simulink model "MotorModelVariable"  (R2016b)
settings: Solver=VariableStepAuto  StartTime=0.0  StopTime=10.0  RelTol=1e-3  EnableMultiTasking=on
undefined symbols (not defined in the file or in its folder): Initial, Motor, Uav
settings Model: Creator=jban039  LastModifiedBy=jban039
settings DataIOCC: LimitDataPoints=on
settings OptimizationCC: LifeSpan=inf
settings DebuggingCC: AllowSymbolicDim=off  SFUnexpectedBacktrackingDiag=warning  SFNoUnconditionalDefaultTransitionDiag=warning  SFExecutionAtInitializationDiag=none
settings ModelReferenceCC: PropagateSignalLabelsOutOfModel=off
settings GRTTargetCC: TargetLangStandard=C89/C90 (ANSI)
settings ConfigComp: CovMetricSettings=dw  CovHtmlReporting=on  CovSaveCumulativeToWorkspaceVar=on  CovSaveSingleToWorkspaceVar=on  CovExternalEMLEnable=off

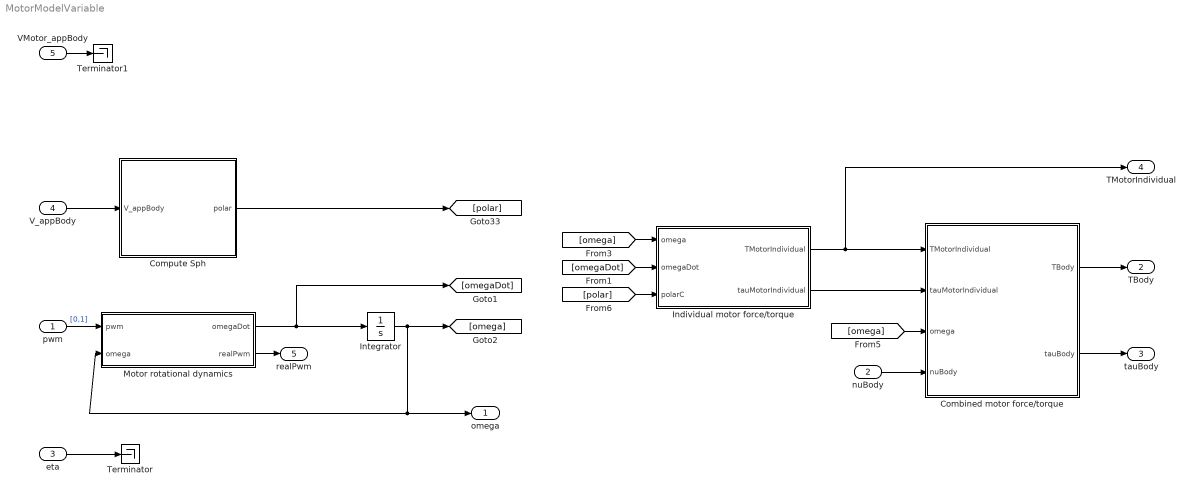
== system MotorModelVariable ==
  pwm : Inport  PortDimensions=Uav.N_ROTORS
  nuBody : Inport  Port=2  Unit=rad/s  PortDimensions=3
  eta : Inport  Port=3  Unit=rad  PortDimensions=3
  V_appBody : Inport  Port=4  Unit=m/s  PortDimensions=3
  VMotor_appBody : Inport  Port=5  Unit=m/s  PortDimensions=[3,4]
  Combined motor force/torque : MATLAB Function  TreatAsAtomicUnit=on
  Compute Sph : MATLAB Function  TreatAsAtomicUnit=on
  Individual motor force/torque : MATLAB Function  TreatAsAtomicUnit=on
  Integrator : Integrator  InitialCondition=Initial.OMEGA
  Motor rotational dynamics : MATLAB Function  TreatAsAtomicUnit=on
  Terminator : Terminator
  Terminator1 : Terminator
  omega : Outport  Unit=rad/s
  TBody : Outport  Port=2  Unit=N
  tauBody : Outport  Port=3  Unit=N*m
  TMotorIndividual : Outport  Port=4  Unit=N
  realPwm : Outport  Port=5
  wires:
  Combined motor force/torque/2(tauBody) -> tauBody/1
  Combined motor force/torque/1(TBody) -> TBody/1
  pwm/1 -> Motor rotational dynamics/1(pwm)  "[0,1]"
  eta/1 -> Terminator/1
  V_appBody/1 -> Compute Sph/1(V_appBody)
  Individual motor force/torque/2(tauMotorIndividual) -> Combined motor force/torque/2(tauMotorIndividual)
  Motor rotational dynamics/1(omegaDot) -> [omegaDot], Integrator/1
  nuBody/1 -> Combined motor force/torque/4(nuBody)
  Compute Sph/1(polar) -> [polar]
  Individual motor force/torque/1(TMotorIndividual) -> Combined motor force/torque/1(TMotorIndividual), TMotorIndividual/1
  [omegaDot] -> Individual motor force/torque/2(omegaDot)
  Integrator/1 -> [omega], Motor rotational dynamics/2(omega), omega/1
  [omega] -> Individual motor force/torque/1(omega)
  [omega] -> Combined motor force/torque/3(omega)
  [polar] -> Individual motor force/torque/3(polarC)
  Motor rotational dynamics/2(realPwm) -> realPwm/1
  VMotor_appBody/1 -> Terminator1/1

== matlab function MotorModelVariable/Compute Sph ==
  data: V_appBody input; polar output
function polar  = computeSph(V_appBody)
%#codegen

% Convert from polar to spherical coordinates

margin = 0.01;

% if ( ( V_appBody(1) < margin ) && ( V_appBody(3) < margin ) )
%     radius = sqrt( sum( V_appBody.^2 ) );
%     azimuth = 0;
%     elevation = 0;
% else
    [ azimuth, elevation, radius ] = cart2sph( V_appBody(1), V_appBody(2), V_appBody(3) );
% end



polar = [azimuth; elevation; radius];

== matlab function MotorModelVariable/Individual motor force//torque ==
  data: omega input; TMotorIndividual output size=[3 4]; omegaDot input; polarC input; Motor parameter; Uav parameter; tauMotorIndividual output size=[3 4]
function [TMotorIndividual, tauMotorIndividual] = motorIndividual( ...
    omega, omegaDot, polarC, Motor, Uav)
%#codegen

elevation = polarC(2);
windSpeed = polarC(3);

% Make assertions to avoid code generation errors
% assert(Uav.N_ROTORS < 16);
Uav.N_ROTORS = 4;

%% Thrust and differential torque

% Concatenated motor force/torque vectors in respective motor frame
% eg. TMotor = [TMotor1, TMotor2, ..., TMotorN]
% where: - N is the number of rotors
%        - TMotorx (x ∈ [1,2,...,N]) is the thrust generated by motor x in
%          its own frame of reference
% TMotorIndividual = [ zeros(2, Uav.N_ROTORS);
%                      K * (omega'.^2) ];

K1 = 6.543988868292138e-05 + ...
     1.886359198743874e-06 * sin(-elevation) + ...
    -7.693938774360465e-07 * windSpeed + ...
     2.639630950517221e-06 * sin(-elevation) * windSpeed + ...
     2.126334444415667e-08 * windSpeed^2;
K2 = -1.903771811601254e-04 + ...
      2.812570127999989e-03 * sin(-elevation) + ...
      1.418616236881443e-03 * windSpeed + ...
     -4.525882966383329e-03 * sin(-elevation) * windSpeed + ...
     -1.658875316836167e-05 * windSpeed^2;

% RECOMPUTE THRUST COEFFICIENTS AS CURRENT VALUES OUT BY FACTOR OF 4
TMotorIndividual = [ zeros(2, Uav.N_ROTORS);
                     0.25 * 0.5 * Uav.RHO_AIR * K1 * (omega'.^2) + ...
                     0.25 * 0.5 * Uav.RHO_AIR * K2 * (omega') ];
tauMotorIndividual = zeros(3, Uav.N_ROTORS);                 
for i = 1:Uav.N_ROTORS
    tauMotorIndividual(:,i) = [ zeros(2, 1);
                               -Uav.ROTOR_DIRECTION(i) .* ...
                               ( Motor.B(i) * (omega(i)'.^2) + Motor.I_R(3,3,i) * omegaDot(i)' ) ];
end

== matlab function MotorModelVariable/Motor rotational dynamics ==
  data: pwm input; omegaDot output; omega input; realPwm output
function [omegaDot, realPwm]  = motorRotDynamics( pwm, omega)
%#codegen

realPwm = (1000 * pwm + 1000);
% realPwm(2) = realPwm(2) - 200;
% realPwm(4) = realPwm(4) - 200;

% realPwm( realPwm < 1230 ) = 1230;

rotorTimeConst = 7.006512e-02;
omegaRef = zeros(4,1);
omegaRef([1 3]) = 0.87*sqrt(0.69)*(7.969173e-1 .* realPwm([1 3]) - 6.528579e2);
omegaRef([2 4]) = 0.87*sqrt(1.31)*(7.969173e-1 .* realPwm([2 4]) - 6.528579e2);
%omegaRef = 7.969173e-1 .* realPwm - 6.528579e2;

omegaDot = (omegaRef - omega) / rotorTimeConst;

== matlab function MotorModelVariable/Combined motor force//torque ==
  data: TMotorIndividual input; TBody output size=3; tauMotorIndividual input; tauBody output size=3; omega input; nuBody input; Motor parameter; Uav parameter
function [TBody, tauBody] = motorCombined( TMotorIndividual,tauMotorIndividual,  ...
    omega, nuBody, Motor, Uav)
%#codegen
assert(Uav.N_ROTORS < 16);

% Initialise matrices to store motor force/torque vectors in body frame
TBodyIndividual   = zeros(3, Uav.N_ROTORS);
tauBodyIndividual = zeros(3, Uav.N_ROTORS);

% Calculate forces and moments from each motor in the body frame
for i = 1:Uav.N_ROTORS
    l = Uav.L(i);
    beta = Uav.BETA(i);
    
    % Matrix to compute torque applied by rotor thrust
 	L = [ 0,            0,            l*sin(beta);
          0,            0,           -l*cos(beta);
         -l*sin(beta),  l*cos(beta),  0 ];

	% Motor force/torque vectors in body frame
	TBodyIndividual(:,i) = Uav.R_MOTOR_TO_BODY(:,:,i) * ...
        TMotorIndividual(:,i);
	tauBodyIndividual(:,i) = Uav.R_MOTOR_TO_BODY(:,:,i) * ...
        tauMotorIndividual(:,i) + L * TBodyIndividual(:,i);
end

%% Gyroscopic moments

% Concatenated gyroscopic moments for each rotor
M_GBodyIndividual = zeros(3, Uav.N_ROTORS);
H_MMotorSeparate = zeros(3, Uav.N_ROTORS);

% Concatenated motor speeds in their respective frames
omegaMotor = [ zeros(2, Uav.N_ROTORS);
               Uav.ROTOR_DIRECTION .* omega' ];

for i = 1:Uav.N_ROTORS
    % Angular momentum in motor frame
    H_MMotorSeparate(:,i) = Motor.I_R(:,:,i) * omegaMotor(:,i);
    % Gyroscopic moment vectors in body frame
    M_GBodyIndividual(:,i) = cross( nuBody, ...
        Uav.R_MOTOR_TO_BODY(:,:,i) * H_MMotorSeparate(:,i) );
end

M_GBody = sum(M_GBodyIndividual, 2);

%% Total torque and moment

% Total force/torque in body frame
TBody = sum(TBodyIndividual, 2);
tauBody = sum(tauBodyIndividual, 2) - M_GBody;

end
